simulink model "board_edit_lab6"  (R2015a)
settings: Solver=ode3  StartTime=0.0  StopTime=inf  FixedStep=0.001  RelTol=1e-3
values from neighbouring files (symbols this model uses):
  A = 0.04    [callback.m]
  frequency = 0.2    [callback.m]
  PID_sim = PID(4)    [callback.m]
  ref_2 = [0 0 ]    [callback.m]
  ref_3 = [0.08 0.06]    [callback.m]
  T1gain = Pt1(1)    [callback.m]
  T1offset = Pt1(2)    [callback.m]
  T2gain = Pt2(1)    [callback.m]
  T2offset = Pt2(2)    [callback.m]
  Xtare_raw = [870 1250 2036 2836 3410]    [callback.m]
  Xtare_real = [-127.5 -80 0 80 127.5] * 1e-3    [callback.m]
  Ytare_raw = [890 1370 2040 2690 3409]    [callback.m]
  Ytare_real = [-97.5 -50 0 50 110]*1e-3    [callback.m]
undefined symbols (not defined in the file or in its folder): Kx, Kxi, Ky, Kyi, ref, V2theta_x, V2theta_y
libraries: PoliArd x12, simulink x4, simulink_extras x1, dspsigops x1
settings Model: ExtModeTrigDuration=2  Creator=User  LastModifiedBy=user
settings OptimizationCC: OptimizeModelRefInitCode=on  LifeSpan=1
settings DebuggingCC: UnderspecifiedInitializationDetection=Classic  MergeDetectMultiDrivingBlocksExec=none
settings HardwareCC: ProdLargestAtomicInteger=Long  ProdLargestAtomicFloat=Double  ProdEndianess=LittleEndian  ProdHWDeviceType=ARM Compatible->ARM Cortex
settings RTWCC: SystemTargetFile=realtime.tlc  GenerateMakefile=off  TemplateMakefile=realtime.tmf  Description=Run on Target Hardware  RTWVerbose=off
settings ERTTargetCC: CombineOutputUpdateFcns=off  ExtModeTransport=3  ExtModeMexFile=ext_serial_win32_comm_rtt  ExtModeMexArgs=0 1 9600  InlinedParameterPlacement=Hierarchical  ERTSrcFileBannerTemplate=realtime_code_template.cgt  ERTHdrFileBannerTemplate=realtime_code_template.cgt  ERTDataSrcFileTemplate=realtime_code_template.cgt  ERTDataHdrFileTemplate=realtime_code_template.cgt  ERTCustomFileTemplate=realtime_file_process.tlc

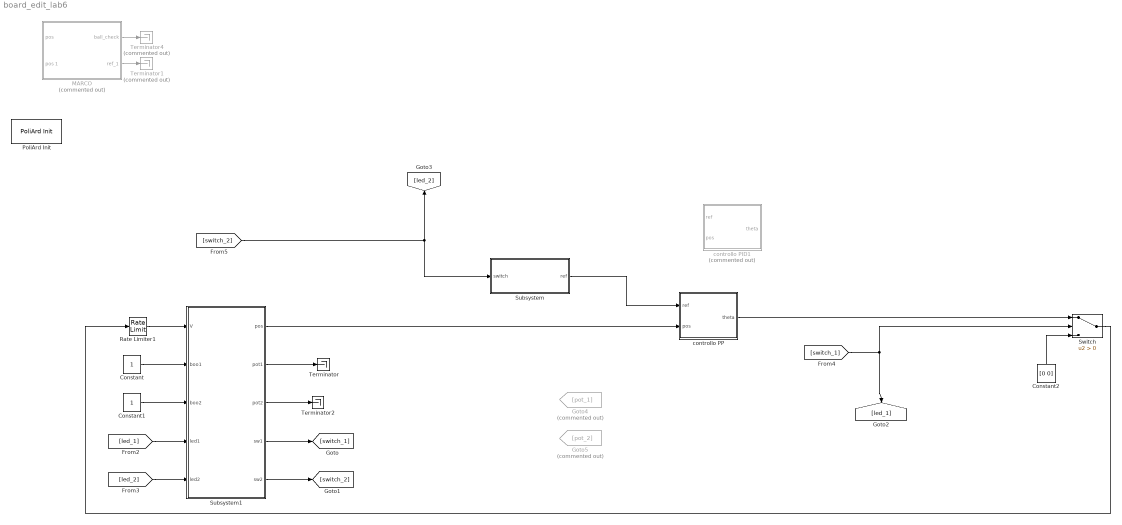
== system board_edit_lab6 ==
  Constant : Constant  OutDataTypeStr=boolean  SampleTime=0.01
  Constant1 : Constant  OutDataTypeStr=boolean  SampleTime=0.01
  Constant2 : Constant  Value=[0 0]  SampleTime=0.01
  Goto4 : Goto  Commented=on  GotoTag=pot_1
  Goto5 : Goto  Commented=on  GotoTag=pot_2
  MARCO : Subsystem  Commented=on
  PoliArd Init : PoliArd/PoliArd Init
  Rate Limiter1 : RateLimiter  RisingSlewLimit=18  FallingSlewLimit=-18  SampleTimeMode=inherited
  Subsystem : Subsystem
  Subsystem1 : Subsystem
  Switch : Switch  Criteria=u2 > Threshold
  Terminator : Terminator
  Terminator1 : Terminator  Commented=on
  Terminator2 : Terminator
  Terminator4 : Terminator  Commented=on
  controllo PID1 : Subsystem  Commented=on  SystemSampleTime=0.01
  "controllo PP " : Subsystem  SystemSampleTime=0.01
  wires:
  Subsystem1/1("pos ") -> "controllo PP "/2("pos ")
  Subsystem1/4(sw1) -> [switch_1]
  Subsystem1/5(sw2) -> [switch_2]
  [led_1] -> Subsystem1/4("led1 ")
  Constant/1 -> Subsystem1/2(boo1)
  Constant1/1 -> Subsystem1/3(boo2)
  [led_2] -> Subsystem1/5(led2)
  MARCO/2(ref_1) -> Terminator1/1
  [switch_1] -> Switch/2, [led_1]
  MARCO/1(ball_check) -> Terminator4/1
  Constant2/1 -> Switch/3
  "controllo PP "/1(theta) -> Switch/1
  Switch/1 -> Rate Limiter1/1
  Rate Limiter1/1 -> Subsystem1/1(V)
  Subsystem1/3(pot2) -> Terminator2/1
  Subsystem1/2(pot1) -> Terminator/1
  [switch_2] -> [led_2], Subsystem/1("switch ")
  Subsystem/1("ref ") -> "controllo PP "/1("ref ")

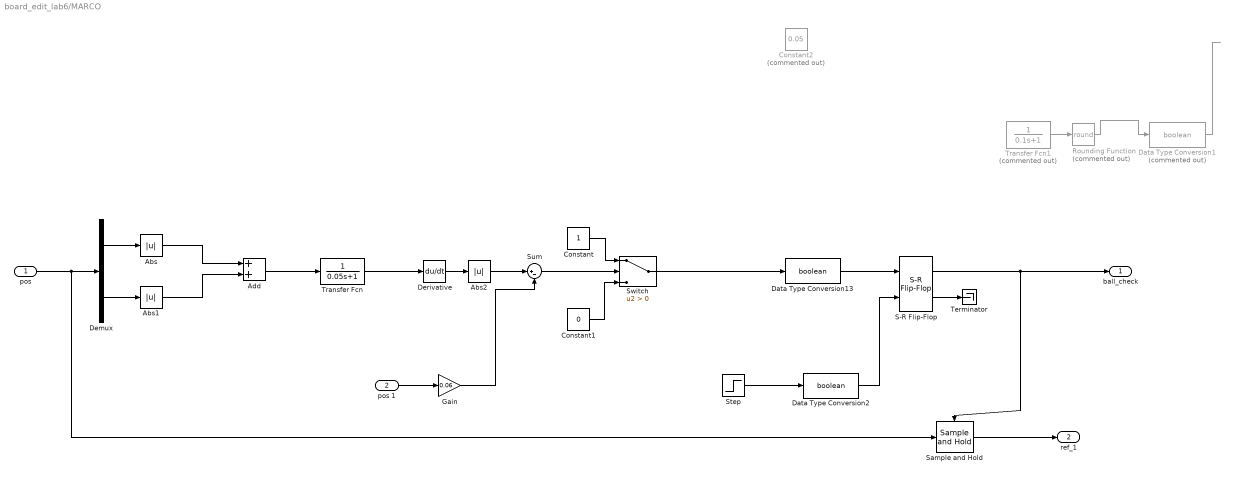
== system board_edit_lab6/MARCO ==
  "pos " : Inport
  pos 1 : Inport  Port=2
  Abs : Abs
  Abs1 : Abs
  Abs2 : Abs
  Add : Sum
  Constant : Constant
  Constant1 : Constant  Value=0
  Constant2 : Constant  Commented=on  Value=0.05
  Data Type Conversion1 : DataTypeConversion  Commented=on  OutDataTypeStr=boolean
  Data Type Conversion13 : DataTypeConversion  OutDataTypeStr=boolean
  Data Type Conversion2 : DataTypeConversion  OutDataTypeStr=boolean
  Demux : Demux  Outputs=2
  Derivative : Derivative
  Gain : Gain  Gain=0.06
  Rounding Function : Rounding  Commented=on  Operator=round
  S-R Flip-Flop : simulink_extras/Flip Flops/S-R Flip-Flop  initial_condition=0
  Sample and Hold : dspsigops/Sample and Hold  trig=Rising edge  initCond=0  latchinput=off
  Step : Step  Before=1  After=0
  Sum : Sum  Inputs=|+-
  Switch : Switch  Criteria=u2 > Threshold
  Terminator : Terminator
  Transfer Fcn : TransferFcn  Denominator=[0.05 1]
  Transfer Fcn1 : TransferFcn  Commented=on  Denominator=[0.1 1]
  ball_check : Outport
  ref_1 : Outport  Port=2
  wires:
  "pos "/1 -> Sample and Hold/1, Demux/1
  Demux/1 -> Abs/1
  Demux/2 -> Abs1/1
  Abs1/1 -> Add/2
  Abs/1 -> Add/1
  Derivative/1 -> Abs2/1
  Abs2/1 -> Sum/1
  Sum/1 -> Switch/2
  Constant/1 -> Switch/1
  Constant1/1 -> Switch/3
  Sample and Hold/1 -> ref_1/1
  Add/1 -> Transfer Fcn/1
  Transfer Fcn/1 -> Derivative/1
  Gain/1 -> Sum/2
  S-R Flip-Flop/1 -> ball_check/1, Sample and Hold/Trigger
  S-R Flip-Flop/2 -> Terminator/1
  Data Type Conversion13/1 -> S-R Flip-Flop/1
  Switch/1 -> Data Type Conversion13/1
  Transfer Fcn1/1 -> Rounding Function/1
  Rounding Function/1 -> Data Type Conversion1/1
  ? -> Transfer Fcn1/1
  Data Type Conversion1/1 -> ?
  Data Type Conversion2/1 -> S-R Flip-Flop/2
  Step/1 -> Data Type Conversion2/1
  pos 1/1 -> Gain/1

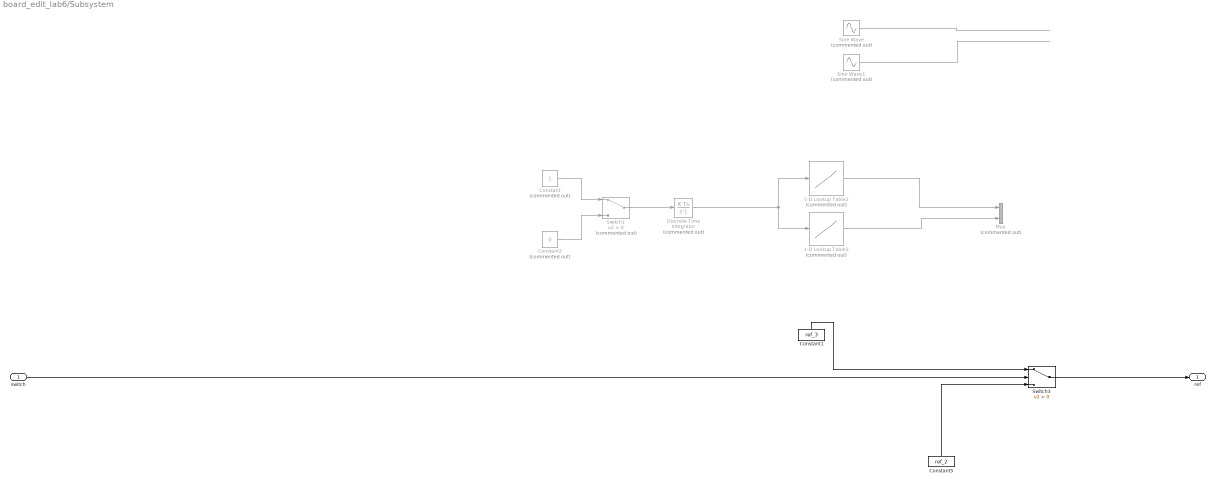
== system board_edit_lab6/Subsystem ==
  "switch " : Inport
  1-D Lookup Table2 : Lookup_n-D  Commented=on  NumberOfTableDimensions=1  BreakpointsForDimension1=ref.x.t  Table=ref.x.v  InternalRulePriority=Speed  RndMeth=Simplest  InputSameDT=on
  1-D Lookup Table3 : Lookup_n-D  Commented=on  NumberOfTableDimensions=1  BreakpointsForDimension1=ref.y.t  Table=ref.y.v  InternalRulePriority=Speed  RndMeth=Simplest  InputSameDT=on
  Constant : Constant  Commented=on  SampleTime=-1
  Constant1 : Constant  Value=ref_3  SampleTime=0.01
  Constant2 : Constant  Commented=on  Value=0  SampleTime=-1
  Constant5 : Constant  Value=ref_2  SampleTime=0.01
  Discrete-Time Integrator : DiscreteIntegrator  Commented=on  gainval=1  InitialConditionSetting=State (most efficient)  SampleTime=0.01  LimitOutput=on
  Mux : Mux  Commented=on  Inputs=2
  Sine Wave : Sin  Commented=on  TimeSource=Use external signal  Amplitude=A  Frequency=frequency*2*pi  SampleTime=0
  Sine Wave1 : Sin  Commented=on  TimeSource=Use external signal  Amplitude=A  Frequency=frequency * 2 * pi  Phase=pi/2  SampleTime=0
  Switch1 : Switch  Commented=on  Criteria=u2 > Threshold
  Switch3 : Switch  Criteria=u2 > Threshold
  "ref " : Outport
  wires:
  Constant5/1 -> Switch3/3
  Switch3/1 -> "ref "/1
  "switch "/1 -> Switch3/2
  Constant/1 -> Switch1/1
  Constant2/1 -> Switch1/3
  Switch1/1 -> Discrete-Time Integrator/1
  Sine Wave1/1 -> ?
  Sine Wave/1 -> ?
  1-D Lookup Table3/1 -> Mux/2
  1-D Lookup Table2/1 -> Mux/1
  Discrete-Time Integrator/1 -> 1-D Lookup Table2/1, 1-D Lookup Table3/1
  Constant1/1 -> Switch3/1

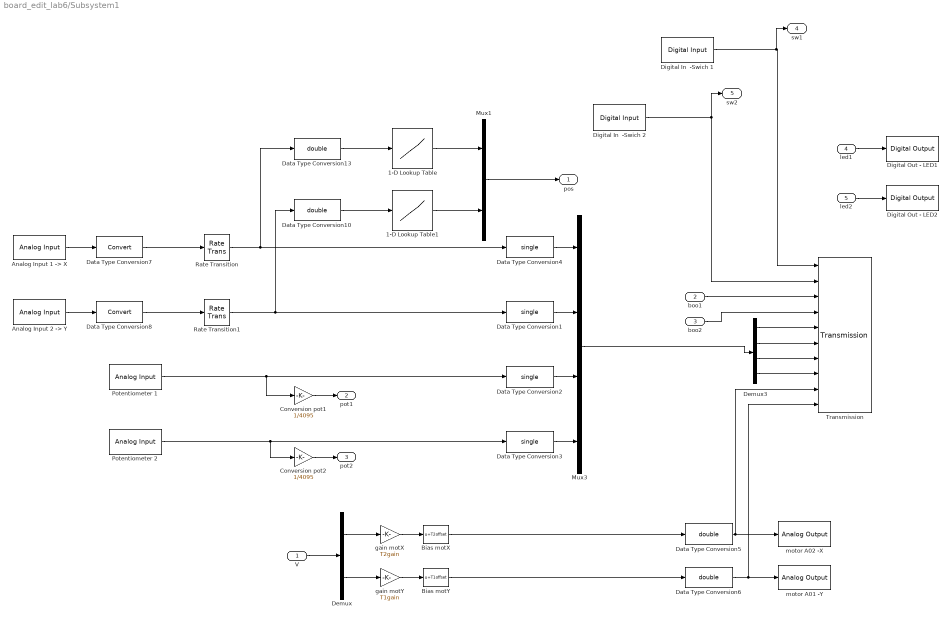
== system board_edit_lab6/Subsystem1 ==
  V : Inport
  boo1 : Inport  Port=2
  boo2 : Inport  Port=3
  "led1 " : Inport  Port=4
  led2 : Inport  Port=5
  1-D Lookup Table : Lookup_n-D  NumberOfTableDimensions=1  BreakpointsForDimension1=Xtare_raw  Table=Xtare_real  InternalRulePriority=Speed  RndMeth=Simplest  InputSameDT=on
  1-D Lookup Table1 : Lookup_n-D  NumberOfTableDimensions=1  BreakpointsForDimension1=Ytare_raw  Table=Ytare_real  InternalRulePriority=Speed  RndMeth=Simplest  InputSameDT=on
  "Analog Input 1 -> X" : PoliArd/Analog Input  AIpin_mask=1  AIsample=0.01
  "Analog Input 2 -> Y" : PoliArd/Analog Input  AIpin_mask=2  AIsample=0.01
  Bias motX : Bias  Bias=T2offset
  Bias motY : Bias  Bias=T1offset
  Conversion pot1 : Gain  Gain=1/4095
  Conversion pot2 : Gain  Gain=1/4095
  Data Type Conversion{1..4} (4 alike) : DataTypeConversion  OutDataTypeStr=single
  Data Type Conversion{5..6,10,13} (4 alike) : DataTypeConversion  OutDataTypeStr=double
  Data Type Conversion7 : DataTypeConversion
  Data Type Conversion8 : DataTypeConversion
  Demux : Demux  Outputs=2
  Demux3 : Demux
  Digital In  -Swich 1 : PoliArd/Digital Input  DI_pin=2  DIsample=0.01
  Digital In  -Swich 2 : PoliArd/Digital Input  DI_pin=3  DIsample=0.01
  Digital Out - LED1 : PoliArd/Digital Output  DO_pin=1
  Digital Out - LED2 : PoliArd/Digital Output  DO_pin=2
  Mux1 : Mux  Inputs=2
  Mux3 : Mux
  Potentiometer 1 : PoliArd/Analog Input  AIpin_mask=8  AIsample=-1
  Potentiometer 2 : PoliArd/Analog Input  AIpin_mask=9  AIsample=-1
  Rate Transition : RateTransition  OutPortSampleTime=0.01
  Rate Transition1 : RateTransition  OutPortSampleTime=0.01
  Transmission : PoliArd/Transmission  sample_freq=100  sig_to_send=6
  gain motX : Gain  Gain=T2gain
  gain motY : Gain  Gain=T1gain
  motor A01 -Y : PoliArd/Analog Output  DAC_pin_mask=2
  motor A02 -X : PoliArd/Analog Output  DAC_pin_mask=1
  "pos " : Outport
  pot1 : Outport  Port=2
  pot2 : Outport  Port=3
  sw1 : Outport  Port=4
  sw2 : Outport  Port=5
  wires:
  Demux3/3 -> Transmission/7
  Demux3/1 -> Transmission/5
  Demux3/2 -> Transmission/6
  Conversion pot2/1 -> pot2/1
  Potentiometer 2/1 -> Data Type Conversion3/1, Conversion pot2/1
  Conversion pot1/1 -> pot1/1
  Potentiometer 1/1 -> Conversion pot1/1, Data Type Conversion2/1
  boo1/1 -> Transmission/3
  boo2/1 -> Transmission/4
  "led1 "/1 -> Digital Out - LED1/1
  led2/1 -> Digital Out - LED2/1
  Mux1/1 -> "pos "/1
  Digital In  -Swich 1/1 -> Transmission/1, sw1/1
  Digital In  -Swich 2/1 -> sw2/1, Transmission/2
  "Analog Input 1 -> X"/1 -> Data Type Conversion7/1
  "Analog Input 2 -> Y"/1 -> Data Type Conversion8/1
  gain motX/1 -> Bias motX/1
  gain motY/1 -> Bias motY/1
  Demux/1 -> gain motX/1
  Demux/2 -> gain motY/1
  V/1 -> Demux/1
  Demux3/4 -> Transmission/8
  Bias motY/1 -> Data Type Conversion6/1
  Data Type Conversion5/1 -> motor A02 -X/1, Transmission/9
  Data Type Conversion6/1 -> Transmission/10, motor A01 -Y/1
  Bias motX/1 -> Data Type Conversion5/1
  Data Type Conversion13/1 -> 1-D Lookup Table/1
  1-D Lookup Table/1 -> Mux1/1
  Data Type Conversion10/1 -> 1-D Lookup Table1/1
  1-D Lookup Table1/1 -> Mux1/2
  Mux3/1 -> Demux3/1
  Data Type Conversion4/1 -> Mux3/1
  Data Type Conversion1/1 -> Mux3/2
  Data Type Conversion2/1 -> Mux3/3
  Data Type Conversion3/1 -> Mux3/4
  Data Type Conversion7/1 -> Rate Transition/1
  Data Type Conversion8/1 -> Rate Transition1/1
  Rate Transition/1 -> Data Type Conversion13/1, Data Type Conversion4/1
  Rate Transition1/1 -> Data Type Conversion10/1, Data Type Conversion1/1

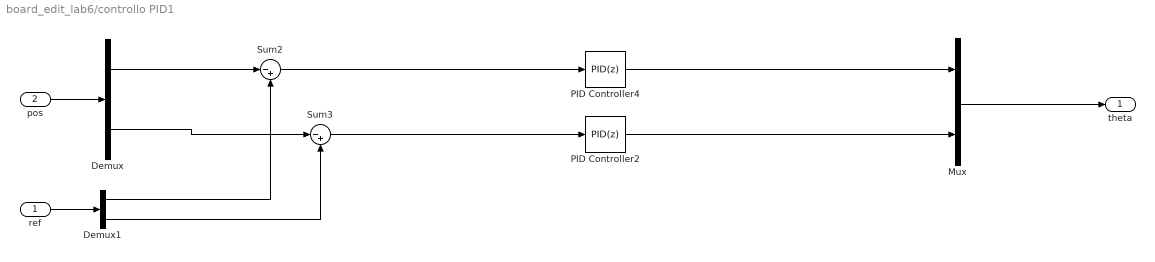
== system board_edit_lab6/controllo PID1 ==
  "ref " : Inport
  "pos " : Inport  Port=2
  Demux : Demux  Outputs=2
  Demux1 : Demux  Outputs=2
  Mux : Mux  Inputs=2
  PID Controller2 : simulink/Continuous/PID Controller  Controller=PID  TimeDomain=Discrete-time  SampleTime=0.01  IntegratorMethod=Forward Euler  FilterMethod=Forward Euler  Form=Parallel  UseFilter=on  ControllerParametersSource=internal  P=PID_sim.y.Kp  I=PID_sim.y.Ki  D=PID_sim.y.Kd  N=PID_sim.y.filter  InitialConditionSource=internal  InitialConditionForIntegrator=0  InitialConditionForFilter=0  ExternalReset=none  LimitOutput=off  UpperSaturationLimit=inf  LowerSaturationLimit=-inf  LinearizeAsGain=on  AntiWindupMode=none  Kb=1  TrackingMode=off  Kt=1  PParamMin=[]  PParamMax=[]  IParamMin=[]  IParamMax=[]  DParamMin=[]  DParamMax=[]  NParamMin=[]  NParamMax=[]  KbParamMin=[]  KbParamMax=[]  KtParamMin=[]  KtParamMax=[]  POutMin=[]  POutMax=[]  IOutMin=[]  IOutMax=[]  DOutMin=[]  DOutMax=[]  NOutMin=[]  NOutMax=[]  KbOutMin=[]  KbOutMax=[]  KtOutMin=[]  KtOutMax=[]  IntegratorOutMin=[]  IntegratorOutMax=[]  FilterOutMin=[]  FilterOutMax=[]  SumOutMin=[]  SumOutMax=[]  SumI1OutMin=[]  SumI1OutMax=[]  SumI2OutMin=[]  SumI2OutMax=[]  SumI3OutMin=[]  SumI3OutMax=[]  SumDOutMin=[]  SumDOutMax=[]  SaturationOutMin=[]  SaturationOutMax=[]  IntegratorContinuousStateAttributes=''  IntegratorStateMustResolveToSignalObject=off  IntegratorRTWStateStorageClass=Auto  FilterContinuousStateAttributes=''  FilterStateMustResolveToSignalObject=off  FilterRTWStateStorageClass=Auto  DifferentiatorICPrevScaledInput=0  DifferentiatorOutMin=[]  DifferentiatorOutMax=[]
  PID Controller4 : simulink/Continuous/PID Controller  Controller=PID  TimeDomain=Discrete-time  SampleTime=0.01  IntegratorMethod=Forward Euler  FilterMethod=Forward Euler  Form=Parallel  UseFilter=on  ControllerParametersSource=internal  P=PID_sim.x.Kp  I=PID_sim.x.Ki  D=PID_sim.x.Kd  N=PID_sim.x.filter  InitialConditionSource=internal  InitialConditionForIntegrator=0  InitialConditionForFilter=0  ExternalReset=none  LimitOutput=off  UpperSaturationLimit=inf  LowerSaturationLimit=-inf  LinearizeAsGain=on  AntiWindupMode=none  Kb=1  TrackingMode=off  Kt=1  PParamMin=[]  PParamMax=[]  IParamMin=[]  IParamMax=[]  DParamMin=[]  DParamMax=[]  NParamMin=[]  NParamMax=[]  KbParamMin=[]  KbParamMax=[]  KtParamMin=[]  KtParamMax=[]  POutMin=[]  POutMax=[]  IOutMin=[]  IOutMax=[]  DOutMin=[]  DOutMax=[]  NOutMin=[]  NOutMax=[]  KbOutMin=[]  KbOutMax=[]  KtOutMin=[]  KtOutMax=[]  IntegratorOutMin=[]  IntegratorOutMax=[]  FilterOutMin=[]  FilterOutMax=[]  SumOutMin=[]  SumOutMax=[]  SumI1OutMin=[]  SumI1OutMax=[]  SumI2OutMin=[]  SumI2OutMax=[]  SumI3OutMin=[]  SumI3OutMax=[]  SumDOutMin=[]  SumDOutMax=[]  SaturationOutMin=[]  SaturationOutMax=[]  IntegratorContinuousStateAttributes=''  IntegratorStateMustResolveToSignalObject=off  IntegratorRTWStateStorageClass=Auto  FilterContinuousStateAttributes=''  FilterStateMustResolveToSignalObject=off  FilterRTWStateStorageClass=Auto  DifferentiatorICPrevScaledInput=0  DifferentiatorOutMin=[]  DifferentiatorOutMax=[]
  Sum2 : Sum  Inputs=|-+
  Sum3 : Sum  Inputs=|-+
  theta : Outport
  wires:
  "ref "/1 -> Demux1/1
  "pos "/1 -> Demux/1
  Mux/1 -> theta/1
  Demux/1 -> Sum2/1
  Demux/2 -> Sum3/1
  Demux1/1 -> Sum2/2
  Demux1/2 -> Sum3/2
  Sum3/1 -> PID Controller2/1
  PID Controller2/1 -> Mux/2
  Sum2/1 -> PID Controller4/1
  PID Controller4/1 -> Mux/1

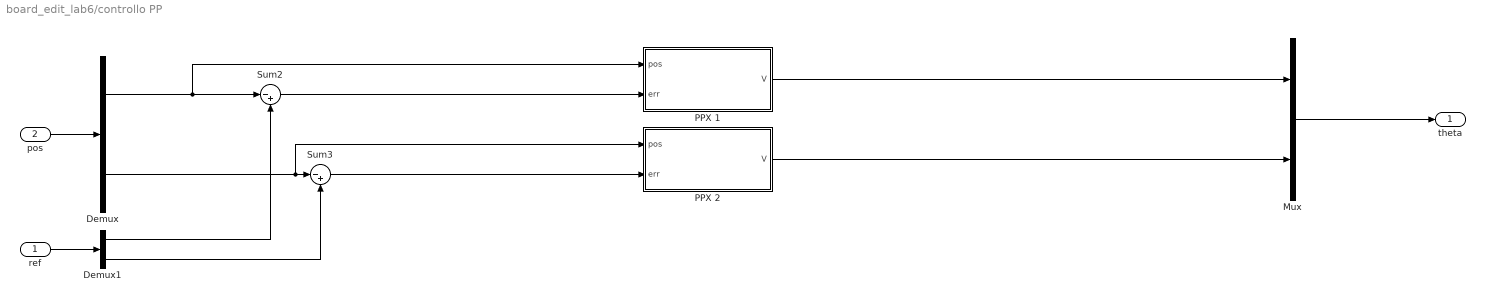
== system board_edit_lab6/controllo PP  ==
  "ref " : Inport
  "pos " : Inport  Port=2
  Demux : Demux  Outputs=2
  Demux1 : Demux  Outputs=2
  Mux : Mux  Inputs=2
  PPX 1 : Subsystem
  PPX 2 : Subsystem
  Sum2 : Sum  Inputs=|-+
  Sum3 : Sum  Inputs=|-+
  theta : Outport
  wires:
  "ref "/1 -> Demux1/1
  "pos "/1 -> Demux/1
  Mux/1 -> theta/1
  Demux/1 -> PPX 1/1("pos "), Sum2/1
  Demux/2 -> PPX 2/1("pos "), Sum3/1
  Demux1/1 -> Sum2/2
  Demux1/2 -> Sum3/2
  Sum3/1 -> PPX 2/2(err)
  Sum2/1 -> PPX 1/2(err)
  PPX 2/1(V) -> Mux/2
  PPX 1/1(V) -> Mux/1

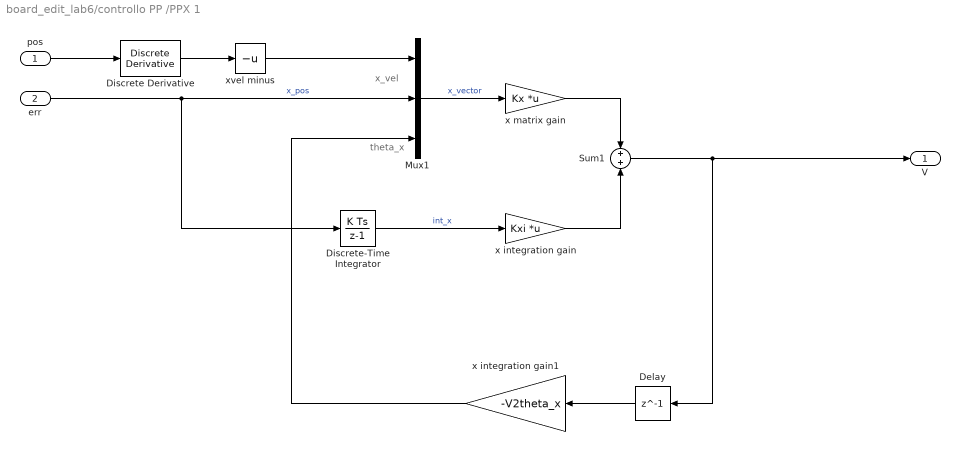
== system board_edit_lab6/controllo PP /PPX 1 ==
  note: theta_x
  note: x_vel
  "pos " : Inport
  err : Inport  Port=2
  Delay : Delay  DelayLength=1  InitialCondition=0
  Discrete Derivative : simulink/Discrete/Discrete Derivative  gainval=1.0  ICPrevScaledInput=0.0  InputProcessing=Inherited  OutMin=[]  OutMax=[]  OutDataType=fixdt(1, 16)  OutScaling=2^-10  DoSatur=off
  Discrete-Time Integrator : DiscreteIntegrator  InitialConditionSetting=State (most efficient)  SampleTime=-1
  Mux1 : Mux  Inputs=3
  Sum1 : Sum  Inputs=+|+
  x integration gain : Gain  Gain=Kxi  Multiplication=Matrix(K*u)
  x integration gain1 : Gain  Gain=-V2theta_x
  x matrix gain : Gain  Gain=Kx  Multiplication=Matrix(K*u)
  xvel minus : UnaryMinus
  V : Outport
  wires:
  x matrix gain/1 -> Sum1/1
  Mux1/1 -> x matrix gain/1  "x_vector"
  x integration gain/1 -> Sum1/2
  Discrete Derivative/1 -> xvel minus/1
  x integration gain1/1 -> Mux1/3
  err/1 -> Discrete-Time Integrator/1, Mux1/2  "x_pos"
  Discrete-Time Integrator/1 -> x integration gain/1  "int_x"
  Sum1/1 -> Delay/1, V/1
  "pos "/1 -> Discrete Derivative/1
  Delay/1 -> x integration gain1/1
  xvel minus/1 -> Mux1/1

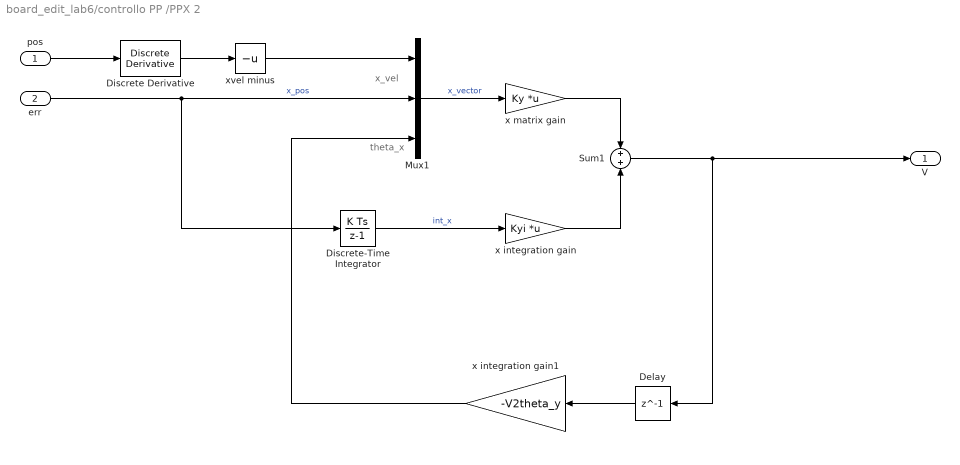
== system board_edit_lab6/controllo PP /PPX 2 ==
  note: theta_x
  note: x_vel
  "pos " : Inport
  err : Inport  Port=2
  Delay : Delay  DelayLength=1  InitialCondition=0
  Discrete Derivative : simulink/Discrete/Discrete Derivative  gainval=1.0  ICPrevScaledInput=0.0  InputProcessing=Inherited  OutMin=[]  OutMax=[]  OutDataType=fixdt(1, 16)  OutScaling=2^-10  DoSatur=off
  Discrete-Time Integrator : DiscreteIntegrator  InitialConditionSetting=State (most efficient)  SampleTime=-1
  Mux1 : Mux  Inputs=3
  Sum1 : Sum  Inputs=+|+
  x integration gain : Gain  Gain=Kyi  Multiplication=Matrix(K*u)
  x integration gain1 : Gain  Gain=-V2theta_y
  x matrix gain : Gain  Gain=Ky  Multiplication=Matrix(K*u)
  xvel minus : UnaryMinus
  V : Outport
  wires:
  x matrix gain/1 -> Sum1/1
  Mux1/1 -> x matrix gain/1  "x_vector"
  x integration gain/1 -> Sum1/2
  Discrete Derivative/1 -> xvel minus/1
  x integration gain1/1 -> Mux1/3
  err/1 -> Discrete-Time Integrator/1, Mux1/2  "x_pos"
  Discrete-Time Integrator/1 -> x integration gain/1  "int_x"
  Sum1/1 -> Delay/1, V/1
  "pos "/1 -> Discrete Derivative/1
  Delay/1 -> x integration gain1/1
  xvel minus/1 -> Mux1/1
